simulink model "MetododeIdentificacionconRele"  (R2021a)
settings: Solver=FixedStepAuto  StartTime=0.0  StopTime=400  FixedStep=1e-3  RelTol=1e-3
settings Model: Creator=Royer  LastModifiedBy=Royer

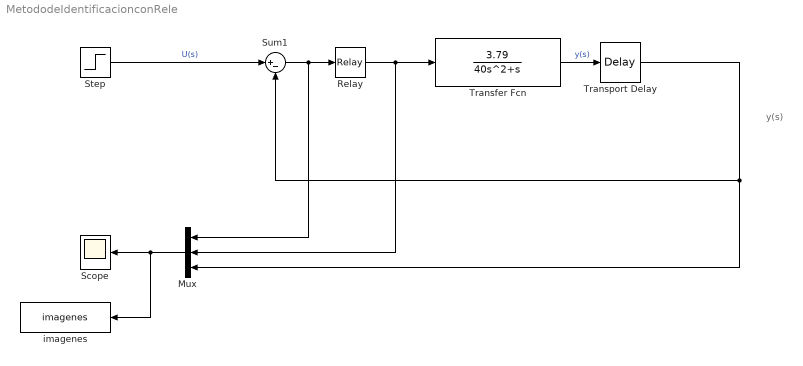
== system MetododeIdentificacionconRele ==
  note: y(s)
  Mux : Mux  Inputs=3
  Relay : Relay  OnSwitchValue=0.25  OffSwitchValue=-0.25  OnOutputValue=0.23  OffOutputValue=-0.30
  Scope : Scope
  Step : Step  Time=0  SampleTime=0
  Sum1 : Sum  Inputs=|+-
  Transfer Fcn : TransferFcn  Numerator=3.79  Denominator=[40 1 0]
  Transport Delay : TransportDelay  DelayTime=2
  imagenes : ToWorkspace  VariableName=imagenes  SaveFormat=Timeseries  SampleTime=-1
  wires:
  Transfer Fcn/1 -> Transport Delay/1  "y(s)"
  Step/1 -> Sum1/1  "U(s)"
  Transport Delay/1 -> Mux/3, Sum1/2
  Relay/1 -> Mux/2, Transfer Fcn/1
  Sum1/1 -> Mux/1, Relay/1
  Mux/1 -> imagenes/1, Scope/1
